simulink model "sinulink7_5"  (R2017a)
settings: Solver=VariableStepAuto  StartTime=0.0  StopTime=30  RelTol=1e-3
settings Model: Creator=adi  LastModifiedBy=adi

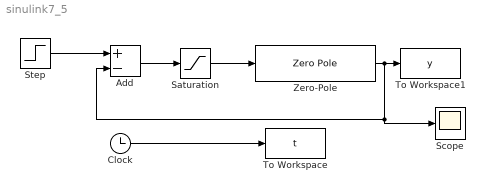
== system sinulink7_5 ==
  Add : Sum  Inputs=+-
  Clock : Clock
      settings: Decimation=30
  Saturation : Saturate  UpperLimit=1  LowerLimit=-1
  Scope : Scope
  Step : Step  Time=0  SampleTime=0
  To Workspace : ToWorkspace  VariableName=t  SampleTime=-1
  To Workspace1 : ToWorkspace  VariableName=y  SampleTime=-1
  Zero-Pole : ZeroPole  Zeros=[]  Poles=[0 -1 -2]  Gain=10
  wires:
  Step/1 -> Add/1
  Saturation/1 -> Zero-Pole/1
  Add/1 -> Saturation/1
  Clock/1 -> To Workspace/1
  Zero-Pole/1 -> Scope/1, Add/2, To Workspace1/1
